simulink model "LQR_and_Trcking_control_fin"  (R2023b)
settings: Solver=VariableStepAuto  StartTime=0.0  StopTime=50.0  RelTol=1e-3
values from neighbouring files (symbols this model uses):
  A = double(A)    [Rotational_inverted_pendulum.m]
  A_uns = double(A_uns)    [Rotational_inverted_pendulum.m]
  B = double(B)    [Rotational_inverted_pendulum.m]
  B_uns = double(B_uns)    [Rotational_inverted_pendulum.m]
  x1_bar = double(sol.x1)    [Rotational_inverted_pendulum.m]
  x1_bar_uns = x1_bar    [Rotational_inverted_pendulum.m]
  x3_bar = 0    [Rotational_inverted_pendulum.m]
  x3_bar_uns = pi    (= 3.14159265359)    [Rotational_inverted_pendulum.m]
undefined symbols (not defined in the file or in its folder): K_lq_track, K_lq_track_uns, K_lq_uns
libraries: simulink_extras x7, simulink x1
settings Model: Creator=Mark  LastModifiedBy=Mark

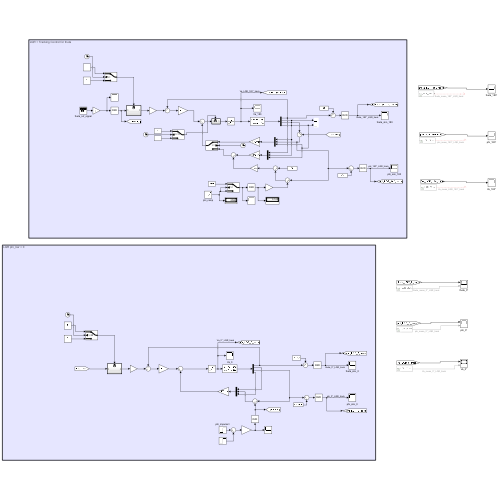
[thumbnail: Simulink's stored preview of the top-level diagram]
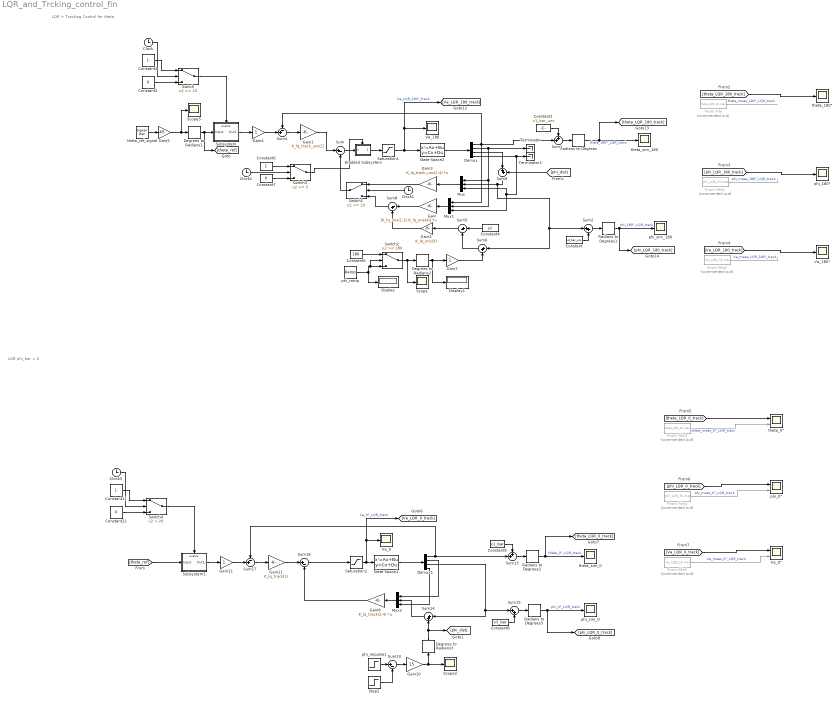
== system LQR_and_Trcking_control_fin ==
  note: LQR + Tracking Control for theta
  note: LQR phi_bar = 0
  Clock{,1..3} (4 alike) : Clock
  Constant : Constant  Value=x3_bar_uns
  Constant1 : Constant  Value=x1_bar_uns
  Constant11 : Constant
  Constant12 : Constant  Value=0
  Constant2 : Constant
  Constant3 : Constant  Value=0
  Constant4 : Constant  Value=pi
  Constant5 : Constant  Value=180
  Constant6 : Constant
  Constant7 : Constant  Value=0
  Constant8 : Constant  Value=x3_bar
  Constant9 : Constant  Value=x1_bar
  Degrees to Radians1 : simulink_extras/Transformations/Degrees to Radians
  Degrees to Radians2 : simulink_extras/Transformations/Degrees to Radians
  Degrees to Radians3 : simulink_extras/Transformations/Degrees to Radians
  Demux : Demux
  Demux1 : Demux
  Display : Display
  Display1 : Display
  Enabled Subsystem : Subsystem  TreatAsAtomicUnit=on
  From File : FromFile  Commented=on  FileName=theta_LQR_32.mat  SampleTime=0
  From File1 : FromFile  Commented=on  FileName=phi_LQR_32.mat  SampleTime=0
  From File2 : FromFile  Commented=on  FileName=Va_LQR_32.mat  SampleTime=0
  From File3 : FromFile  Commented=on  FileName=theta_LQR_35.mat  SampleTime=0
  From File4 : FromFile  Commented=on  FileName=phi_LQR_35.mat  SampleTime=0
  From File5 : FromFile  Commented=on  FileName=Va_LQR_35.mat  SampleTime=0
  Gain : Gain  Gain=[K_lq_uns(1:2) K_lq_uns(4)]  Multiplication=Matrix(K*u) (u vector)
  Gain1 : Gain  Gain=K_lq_track_uns(1)
  Gain10 : Gain  Gain=15
  Gain11 : Gain  Gain=K_lq_track(1)
  Gain12 : Gain
  Gain2 : Gain  Gain=K_lq_uns(3)
  Gain3 : Gain  Gain=K_lq_track_uns(2:4)  Multiplication=Matrix(K*u) (u vector)
  Gain4 : Gain
  Gain5 : Gain  Gain=45
  Gain7 : Gain
  Gain8 : Gain  Gain=K_lq_track(2:4)  Multiplication=Matrix(K*u) (u vector)
  Mux : Mux  Inputs=3
  Mux1 : Mux  Inputs=3
  Mux2 : Mux  Inputs=3
  Radians to Degrees{,1..3} (4 alike) : simulink_extras/Transformations/Radians to Degrees
  Saturation1 : Saturate  UpperLimit=10  LowerLimit=-10
  Saturation2 : Saturate  UpperLimit=10  LowerLimit=-10
  Scope : Scope
  Scope2 : Scope
  Scope3 : Scope
  State-Space1 : StateSpace  A=A  B=B  C=eye(4)  D=zeros(4,1)  InitialCondition=[0 0 0 0]
  State-Space2 : StateSpace  A=A_uns  B=B_uns  C=eye(4)  D=zeros(4,1)  InitialCondition=[0 0 0 0]
  Step2 : Step  Time=20.05  SampleTime=0
  Subsystem : Subsystem
  Subsystem1 : Subsystem
  Sum{,5,10,16} (4 alike) : Sum  Inputs=|+-
  Sum1 : Sum  Inputs=++|
  Sum13 : Sum  Inputs=++|
  Sum{2,6,9,14..15} (5 alike) : Sum  Inputs=|++
  Sum17 : Sum  Inputs=-+|
  Sum4 : Sum  Inputs=-+|
  Sum8 : Sum  Inputs=|-+
  Switch : Switch  Threshold=10  SaturateOnIntegerOverflow=off  InputSameDT=off
  Switch1 : Switch  Threshold=10  SaturateOnIntegerOverflow=off  InputSameDT=off
  Switch2 : Switch  Threshold=180  SaturateOnIntegerOverflow=off  InputSameDT=off
  Switch3 : Switch  Threshold=5  SaturateOnIntegerOverflow=off  InputSameDT=off
  Switch4 : Switch  Criteria=u2 > Threshold  Threshold=20  SaturateOnIntegerOverflow=off  InputSameDT=off
  Terminator : Terminator
  Terminator1 : Terminator
  Va_0 : Scope
  Va_0° : Scope  NumInputPorts=2
  Va_180 : Scope
  Va_180° : Scope
  phi_0° : Scope  NumInputPorts=2
  phi_180° : Scope
  phi_impulse1 : Step  Time=20  SampleTime=0
  phi_ramp : simulink/Sources/Ramp  slope=50  start=0  InitialOutput=0
  phi_sim_0 : Scope
  phi_sim_180 : Scope
  theta_0° : Scope  NumInputPorts=2
  theta_180° : Scope
  theta_ref_signal : SignalGenerator  Frequency=0.05
  theta_sim_0 : Scope
  theta_sim_180 : Scope
  wires:
  Constant/1 -> Sum2/2
  Sum1/1 -> Radians to Degrees/1
  Radians to Degrees1/1 -> [phi_LQR_180_track], phi_sim_180/1  "phi_180°_LQR_track"
  Saturation1/1 -> State-Space2/1, [Va_LQR_180_track], Va_180/1  "Va_LQR_180°_track"
  Demux/1 -> Mux1/1, Sum1/2, Sum4/1
  Constant1/1 -> Sum1/1
  Sum2/1 -> Radians to Degrees1/1
  Switch1/1 -> Sum/2
  Enabled Subsystem/1(Out1) -> Saturation1/1
  State-Space2/1 -> Demux/1
  Radians to Degrees/1 -> [theta_LQR_180_track], theta_sim_180/1  "theta_180°_LQR_track"
  Sum/1 -> Enabled Subsystem/1(In1)
  Demux/2 -> Terminator/1, Mux1/2, Mux/1
  Demux/4 -> Mux1/3, Mux/3, Terminator1/1
  Switch/1 -> Subsystem/Enable
  Constant2/1 -> Switch/1
  Constant3/1 -> Switch/3
  Clock/1 -> Switch/2
  Clock1/1 -> Switch1/2
  Gain3/1 -> Switch1/1
  Sum4/1 -> Gain1/1
  Gain1/1 -> Sum/1
  Subsystem/1(Out1) -> Gain4/1
  Mux/1 -> Gain3/1
  Gain4/1 -> Sum4/2
  theta_ref_signal/1 -> Gain5/1
  Gain5/1 -> Scope3/1, Degrees to Radians1/1
  Degrees to Radians1/1 -> [theta_ref], Subsystem/1(Input)
  Constant5/1 -> Switch2/1
  Degrees to Radians2/1 -> Gain7/1, Display1/1
  Switch2/1 -> Scope/1, Degrees to Radians2/1
  phi_ramp/1 -> Display/1, Switch2/2, Switch2/3
  Sum9/1 -> Mux/2, Sum2/1, Sum6/1
  Constant4/1 -> Sum5/1
  Mux1/1 -> Gain/1
  Gain7/1 -> Sum6/2
  Gain/1 -> Sum8/1
  Constant6/1 -> Switch3/1
  Constant7/1 -> Switch3/3
  Switch3/1 -> Enabled Subsystem/Enable
  Clock2/1 -> Switch3/2
  Sum6/1 -> Sum5/2
  Sum5/1 -> Gain2/1
  Sum8/1 -> Switch1/3
  Gain2/1 -> Sum8/2
  Demux/3 -> Sum9/1
  Mux2/1 -> Gain8/1
  Constant8/1 -> Sum15/2
  Radians to Degrees3/1 -> [phi_LQR_0_track], phi_sim_0/1  "phi_0°_LQR_track"
  phi_impulse1/1 -> Sum10/1
  Sum15/1 -> Radians to Degrees3/1
  Gain10/1 -> Scope2/1, Degrees to Radians3/1
  Step2/1 -> Sum10/2
  Demux1/2 -> Mux2/1
  Saturation2/1 -> Va_0/1, [Va_LQR_0_track], State-Space1/1  "Va_0°_LQR_track"
  Radians to Degrees2/1 -> [theta_LQR_0_track], theta_sim_0/1  "theta_0°_LQR_track"
  Demux1/4 -> Mux2/3
  Degrees to Radians3/1 -> Sum14/2, [phi_dist]
  Demux1/1 -> Sum13/2, Sum17/1
  Constant9/1 -> Sum13/1
  State-Space1/1 -> Demux1/1
  Demux1/3 -> Sum14/1, Sum15/1
  Sum16/1 -> Saturation2/1
  Sum13/1 -> Radians to Degrees2/1
  Sum14/1 -> Mux2/2
  Sum10/1 -> Gain10/1
  Gain8/1 -> Sum16/2
  Constant12/1 -> Switch4/3
  Clock3/1 -> Switch4/2
  Switch4/1 -> Subsystem1/Enable
  Sum17/1 -> Gain11/1
  Gain12/1 -> Sum17/2
  Gain11/1 -> Sum16/1
  Constant11/1 -> Switch4/1
  Subsystem1/1(Out1) -> Gain12/1
  [theta_ref] -> Subsystem1/1(Input)
  [phi_dist] -> Sum9/2
  [theta_LQR_0_track] -> theta_0°/1
  [phi_LQR_0_track] -> phi_0°/1
  [Va_LQR_0_track] -> Va_0°/1
  [theta_LQR_180_track] -> theta_180°/1
  [phi_LQR_180_track] -> phi_180°/1
  [Va_LQR_180_track] -> Va_180°/1
  From File2/1 -> ?  "Va_meas_LQR_180°_track"
  From File1/1 -> ?  "phi_meas_180°_LQR_track"
  From File/1 -> ?  "theta_meas_180°_LQR_track"
  From File3/1 -> theta_0°/2  "theta_meas_0°_LQR_track"
  From File4/1 -> phi_0°/2  "phi_meas_0°_LQR_track"
  From File5/1 -> Va_0°/2  "Va_meas_0°_LQR_track"

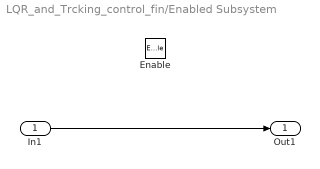
== system LQR_and_Trcking_control_fin/Enabled Subsystem ==
  In1 : Inport
  Enable : EnablePort
  Out1 : Outport
  wires:
  In1/1 -> Out1/1

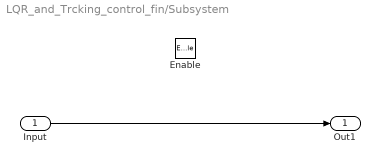
== system LQR_and_Trcking_control_fin/Subsystem ==
  Input : Inport
  Enable : EnablePort
  Out1 : Outport
  wires:
  Input/1 -> Out1/1

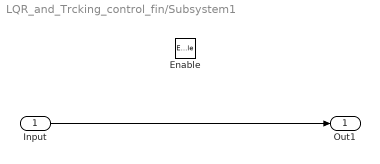
== system LQR_and_Trcking_control_fin/Subsystem1 ==
  Input : Inport
  Enable : EnablePort
  Out1 : Outport
  wires:
  Input/1 -> Out1/1
